simulink model "unicycle_simulink_const_input"  (R2020b)
settings: Solver=VariableStepAuto  StartTime=0.0  StopTime=50  RelTol=1e-3
values from neighbouring files (symbols this model uses):
  Current_coordinates = Target_coordinates    [checking_simulink_with_matlab.m]    (also in lloyd_wtd_adaptive_nonconvex.m = [Prev_Px(i); Prev_Py(i)]; lloyd_wtd_unicycle.m = [Prev_Px(i); Prev_Py(i)])
  init_heading = b(end)    [checking_simulink_with_matlab.m]    (also in lloyd_wtd_adaptive_nonconvex.m = init_heading_list(i); lloyd_wtd_unicycle.m = init_heading_list(i))
  Target_coordinates = [round(rand(1)*10);round(rand(1)*10) ]    [checking_simulink_with_matlab.m]    (also in lloyd_wtd_adaptive_nonconvex.m = [Px(i);Py(i)]; lloyd_wtd_unicycle.m = [Px(i);Py(i)])
libraries: simulink x3, robotmobilelib x1
settings Model: Creator=nijil  LastModifiedBy=nijil

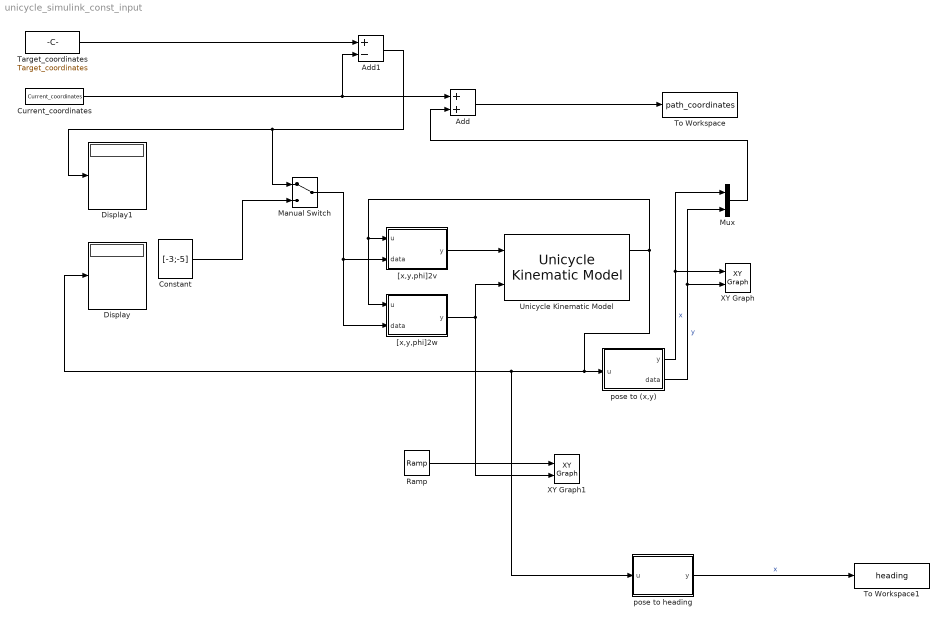
== system unicycle_simulink_const_input ==
  Add : Sum
  Add1 : Sum  Inputs=+-
  Constant : Constant  Value=[-3;-5]  VectorParams1D=off
  Current_coordinates : Constant  Value=Current_coordinates
  Display : Display
  Display1 : Display
  Manual Switch : ManualSwitch
  Mux : Mux  Inputs=2
  Ramp : simulink/Sources/Ramp  slope=1  start=0  InitialOutput=0
  Target_coordinates : Constant  Value=Target_coordinates
  To Workspace : ToWorkspace  VariableName=path_coordinates  SaveFormat=Timeseries  SampleTime=-1
  To Workspace1 : ToWorkspace  VariableName=heading  SaveFormat=Timeseries  SampleTime=-1
  Unicycle Kinematic Model : robotmobilelib/Unicycle Kinematic Model  VehicleInputs=Vehicle Speed & Heading Angular Velocity  WheelRadius=0.1  WheelSpeedRange=[-pi pi]  InitialState=[0 0 init_heading]  SimulateUsing=Interpreted execution
      settings: SourceProductBaseCode=RO
  XY Graph : simulink/Sinks/XY Graph  xmin=-10  xmax=10  ymin=-10  ymax=10  st=-1
  XY Graph1 : simulink/Sinks/XY Graph  xmin=0  xmax=50  ymin=-10  ymax=10  st=-1
  "[x,y,phi]2v" : MATLAB Function  TreatAsAtomicUnit=on
  "[x,y,phi]2w" : MATLAB Function  TreatAsAtomicUnit=on
  pose to (x,y) : MATLAB Function  TreatAsAtomicUnit=on
  pose to heading : MATLAB Function  TreatAsAtomicUnit=on
  wires:
  Ramp/1 -> XY Graph1/1
  "[x,y,phi]2v"/1(y) -> Unicycle Kinematic Model/1
  "[x,y,phi]2w"/1(y) -> XY Graph1/2, Unicycle Kinematic Model/2
  Mux/1 -> Add/2
  Target_coordinates/1 -> Add1/1
  pose to (x,y)/1(y) -> Mux/1, XY Graph/1  "x"
  pose to (x,y)/2(data) -> XY Graph/2, Mux/2  "y"
  Current_coordinates/1 -> Add/1, Add1/2
  Add/1 -> To Workspace/1
  Manual Switch/1 -> "[x,y,phi]2v"/2(data), "[x,y,phi]2w"/2(data)
  pose to heading/1(y) -> To Workspace1/1  "x"
  Unicycle Kinematic Model/1 -> "[x,y,phi]2w"/1(u), "[x,y,phi]2v"/1(u), pose to (x,y)/1(u), pose to heading/1(u), Display/1
  Constant/1 -> Manual Switch/2
  Add1/1 -> Display1/1, Manual Switch/1

== matlab function unicycle_simulink_const_input/[x,y,phi]2v ==
  data: u input; y output; data input
function y = fcn(u, data)
fd=[data(1)-u(1) data(2)-u(2)];
hi=[cos(u(3)) sin(u(3))];
% hip=[-sin(u(3)) cos(u(3))];
y =norm(hi.*(hi*fd'),2);

== matlab function unicycle_simulink_const_input/pose to (x,y) ==
  data: u input; y output; data output
function [y,data] = fcn(u)
y=u(1);
data = u(2);

== matlab function unicycle_simulink_const_input/pose to heading ==
  data: u input; y output
function y = fcn(u)

y = u(3);

== matlab function unicycle_simulink_const_input/[x,y,phi]2w ==
  data: u input; y output; data input
function y = fcn(u, data)
fd=[data(1)-u(1) data(2)-u(2)];
% hi=[cos(u(3)) sin(u(3))];
hip=[-sin(u(3)) cos(u(3))];
y =2*(hip*fd');
